simulink model "Velocity_LQR"  (R2018a)
settings: Solver=VariableStepAuto  StartTime=0.0  StopTime=10.0  MaxStep=1e-2  RelTol=1e-5
PreLoadFcn:
  | modelDir = fileparts(get_param(bdroot, 'FileName'));
  | addpath(fullfile(modelDir,'../../Parameters'));
  | addpath(fullfile(modelDir,'../../Controllers/VelocityLQR'));
  | addpath(fullfile(modelDir,'../../Controllers/VelocityLQR/generated'));
  | 
  | Constants_Kugle
  | Constants_nominal
  | 
  | Parameters_Controllers
  | load('VelocityLQRgain.mat');
InitFcn:
  | Constants_Kugle
  | Constants_nominal
  | 
  | Parameters_Controllers
  | load('VelocityLQRgain.mat');
undefined symbols (not defined in the file or in its folder): Ts, VelocityController_StabilizationDetectionVelocity, VelocityLQR_IntegralEnabled, VelocityLQR_IntegratorPowerupStabilizeTime, VelocityLQR_MaximumKickinVelocity, VelocityLQR_PositionControlAtZeroVelocityReference, VelocityLQRgain, x_init
libraries: qlib x1
settings Model: Creator=thomas  LastModifiedBy=Thomas

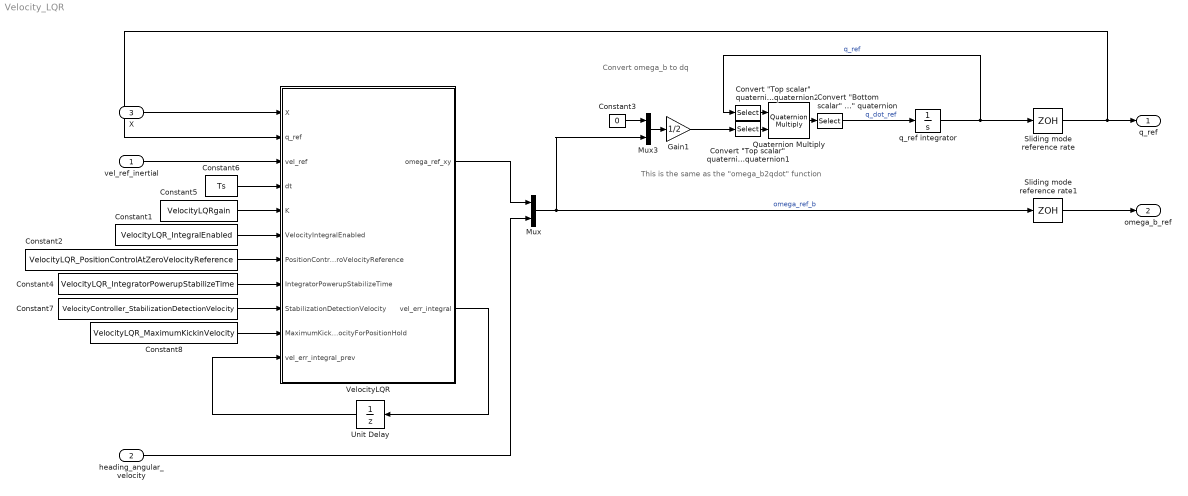
== system Velocity_LQR ==
  note: Convert omega_b to dq
  note: This is the same as the "omega_b2qdot" function
  vel_ref_inertial : Inport  PortDimensions=2
  heading_angular_velocity : Inport  Port=2  PortDimensions=1
  X : Inport  Port=3  PortDimensions=12
  Constant1 : Constant  Value=VelocityLQR_IntegralEnabled  SampleTime=-1
  Constant2 : Constant  Value=VelocityLQR_PositionControlAtZeroVelocityReference  SampleTime=-1
  Constant3 : Constant  Value=0
  Constant4 : Constant  Value=VelocityLQR_IntegratorPowerupStabilizeTime  SampleTime=-1
  Constant5 : Constant  Value=VelocityLQRgain  SampleTime=-1
  Constant6 : Constant  Value=Ts  SampleTime=-1
  Constant7 : Constant  Value=VelocityController_StabilizationDetectionVelocity  SampleTime=-1
  Constant8 : Constant  Value=VelocityLQR_MaximumKickinVelocity  SampleTime=-1
  "Convert \"Bottom scalar\" quaternion to \"Top scalar\" quaternion" : Selector  InputPortWidth=4  IndexOptions=Index vector (dialog)  Indices=[4 1 2 3]  OutputSizes=1
  "Convert \"Top scalar\" quaternion to \"Bottom scalar\" quaternion1" : Selector  InputPortWidth=4  IndexOptions=Index vector (dialog)  Indices=[2 3 4 1]  OutputSizes=1
  "Convert \"Top scalar\" quaternion to \"Bottom scalar\" quaternion2" : Selector  InputPortWidth=4  IndexOptions=Index vector (dialog)  Indices=[2 3 4 1]  OutputSizes=1
  Gain1 : Gain  Gain=1/2
  Mux : Mux  Inputs=2
  Mux3 : Mux  Inputs=2
  Quaternion Multiply : qlib/Quaternion Multiply
  Sliding mode reference rate : ZeroOrderHold  SampleTime=Ts
  Sliding mode reference rate1 : ZeroOrderHold  SampleTime=Ts
  Unit Delay : UnitDelay  InitialCondition=[0;0]  SampleTime=Ts
  VelocityLQR : MATLAB Function  TreatAsAtomicUnit=on  SystemSampleTime=Ts
      settings: MinAlgLoopOccurrences=on
  q_ref integrator : Integrator  InitialCondition=x_init(3:6)
  q_ref : Outport
  omega_b_ref : Outport  Port=2
  wires:
  Constant5/1 -> VelocityLQR/5(K)
  Constant6/1 -> VelocityLQR/4(dt)
  X/1 -> VelocityLQR/1(X)
  Sliding mode reference rate/1 -> VelocityLQR/2(q_ref), q_ref/1
  vel_ref_inertial/1 -> VelocityLQR/3(vel_ref)
  VelocityLQR/2(vel_err_integral) -> Unit Delay/1
  Unit Delay/1 -> VelocityLQR/11(vel_err_integral_prev)
  VelocityLQR/1(omega_ref_xy) -> Mux/1
  Constant2/1 -> VelocityLQR/7(PositionControlAtZeroVelocityReference)
  Constant1/1 -> VelocityLQR/6(VelocityIntegralEnabled)
  Quaternion Multiply/1 -> "Convert \"Bottom scalar\" quaternion to \"Top scalar\" quaternion"/1
  Mux/1 -> Mux3/2, Sliding mode reference rate1/1  "omega_ref_b"
  Mux3/1 -> Gain1/1
  Gain1/1 -> "Convert \"Top scalar\" quaternion to \"Bottom scalar\" quaternion1"/1
  "Convert \"Top scalar\" quaternion to \"Bottom scalar\" quaternion1"/1 -> Quaternion Multiply/2
  Constant3/1 -> Mux3/1
  "Convert \"Bottom scalar\" quaternion to \"Top scalar\" quaternion"/1 -> q_ref integrator/1  "q_dot_ref"
  q_ref integrator/1 -> "Convert \"Top scalar\" quaternion to \"Bottom scalar\" quaternion2"/1, Sliding mode reference rate/1  "q_ref"
  "Convert \"Top scalar\" quaternion to \"Bottom scalar\" quaternion2"/1 -> Quaternion Multiply/1
  Sliding mode reference rate1/1 -> omega_b_ref/1
  heading_angular_velocity/1 -> Mux/2
  Constant4/1 -> VelocityLQR/8(IntegratorPowerupStabilizeTime)
  Constant7/1 -> VelocityLQR/9(StabilizationDetectionVelocity)
  Constant8/1 -> VelocityLQR/10(MaximumKickinVelocityForPositionHold)

== matlab function Velocity_LQR/VelocityLQR ==
  data: X input size=12; q_ref input size=4; vel_ref input size=2; dt input; K input; VelocityIntegralEnabled input; PositionControlAtZeroVelocityReference input; IntegratorPowerupStabilizeTime input; StabilizationDetectionVelocity input; MaximumKickinVelocityForPositionHold input; vel_err_integral_prev input; omega_ref_xy output size=2; vel_err_integral output size=2
function [omega_ref_xy, vel_err_integral] = VelocityLQR_(X, q_ref, vel_ref, dt, K, VelocityIntegralEnabled, PositionControlAtZeroVelocityReference, IntegratorPowerupStabilizeTime, StabilizationDetectionVelocity, MaximumKickinVelocityForPositionHold, vel_err_integral_prev)
    [omega_ref_xy, vel_err_integral] = VelocityLQR(X, q_ref, vel_err_integral_prev, vel_ref, dt, K, VelocityIntegralEnabled, PositionControlAtZeroVelocityReference, IntegratorPowerupStabilizeTime, StabilizationDetectionVelocity, MaximumKickinVelocityForPositionHold);
end
